simulink model "LQR_sim"  (R2025b)
settings: Solver=VariableStepAuto  StartTime=0.0  StopTime=5  RelTol=1e-3
values from neighbouring files (symbols this model uses):
  A = zeros(4,4)    [get_linearized_matrices.m]
  B = zeros(4,1)    [get_linearized_matrices.m]
  bb = params    [LQR_test.m]
  C = diag([1,0,0,0])    [KalmanFilter.m]    (also in get_linearized_matrices.m = eye(4))
  D = zeros(4,1)    [get_linearized_matrices.m]
  ic = [0; 0.175; 0; 0]    [LQR_test.m]
  K = get_gains_LQR_vertical(0)    [bandwidth_test.m]
  ref = [0;0; 1; 0]    [LQR_test.m]
undefined symbols (not defined in the file or in its folder): Kr
settings Model: Creator=JPham  LastModifiedBy=JPham

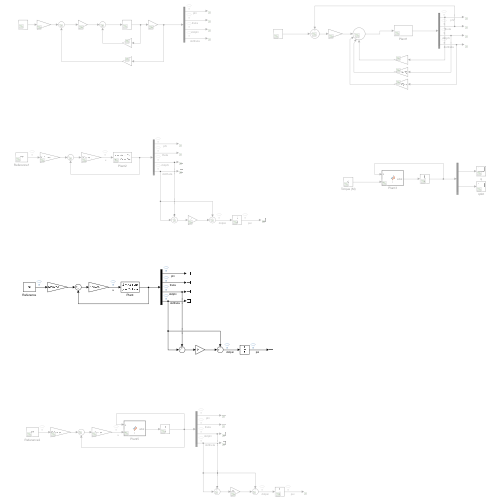
[thumbnail: Simulink's stored preview of the top-level diagram]
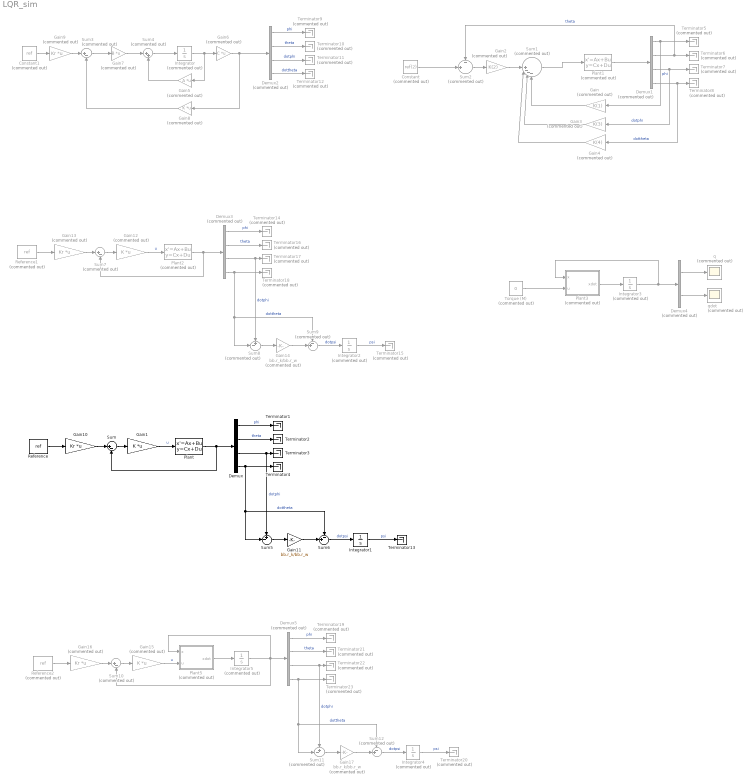
== system LQR_sim ==
  Constant : Constant  Commented=on  Value=ref(2)
  Constant1 : Constant  Commented=on  Value=ref
  Demux : Demux
  Demux{1..3,5} (4 alike) : Demux  Commented=on
  Demux4 : Demux  Commented=on  Outputs=2
  Gain : Gain  Commented=on  Gain=K(1)
  Gain1 : Gain  Gain=K  Multiplication=Matrix(K*u) (u vector)
  Gain10 : Gain  Gain=Kr  Multiplication=Matrix(K*u) (u vector)
  Gain11 : Gain  Gain=bb.r_k/bb.r_w
  Gain12 : Gain  Commented=on  Gain=K  Multiplication=Matrix(K*u) (u vector)
  Gain13 : Gain  Commented=on  Gain=Kr  Multiplication=Matrix(K*u) (u vector)
  Gain14 : Gain  Commented=on  Gain=bb.r_k/bb.r_w
  Gain15 : Gain  Commented=on  Gain=K  Multiplication=Matrix(K*u) (u vector)
  Gain16 : Gain  Commented=on  Gain=Kr  Multiplication=Matrix(K*u) (u vector)
  Gain17 : Gain  Commented=on  Gain=bb.r_k/bb.r_w
  Gain2 : Gain  Commented=on  Gain=K(2)
  Gain3 : Gain  Commented=on  Gain=K(3)
  Gain4 : Gain  Commented=on  Gain=K(4)
  Gain5 : Gain  Commented=on  Gain=A  Multiplication=Matrix(K*u)
  Gain6 : Gain  Commented=on  Gain=C  Multiplication=Matrix(K*u)
  Gain7 : Gain  Commented=on  Gain=B  Multiplication=Matrix(K*u)
  Gain8 : Gain  Commented=on  Gain=K  Multiplication=Matrix(K*u)
  Gain9 : Gain  Commented=on  Gain=Kr  Multiplication=Matrix(K*u)
  Integrator : Integrator  Commented=on  InitialCondition=ic
  Integrator1 : Integrator
  Integrator2 : Integrator  Commented=on
  Integrator3 : Integrator  Commented=on  InitialCondition=[0; 0.3; 0; -1]  ContinuousStateAttributes='angle'
  Integrator4 : Integrator  Commented=on
  Integrator5 : Integrator  Commented=on  InitialCondition=ic  ContinuousStateAttributes='angle'
  Plant : StateSpace  A=A  B=B  C=C  D=D  InitialCondition=ic  ContinuousStateAttributes={'phi', 'theta', 'dot_phi', 'dot_theta'}
  Plant1 : StateSpace  Commented=on  A=A  B=B  C=C  D=D  InitialCondition=ic  ContinuousStateAttributes={'phi', 'theta', 'dot_phi', 'dot_theta'}
  Plant2 : StateSpace  Commented=on  A=A  B=B  C=C  D=D  InitialCondition=ic  ContinuousStateAttributes={'phi', 'theta', 'dot_phi', 'dot_theta'}
  Plant3 : MATLAB Function  Commented=on  TreatAsAtomicUnit=on
  Plant5 : MATLAB Function  Commented=on  TreatAsAtomicUnit=on
  Reference : Constant  Value=ref
  Reference1 : Constant  Commented=on  Value=ref
  Reference2 : Constant  Commented=on  Value=ref
  Sum : Sum  Inputs=|+-
  Sum1 : Sum  Commented=on  Inputs=|||+---
  Sum10 : Sum  Commented=on  Inputs=|+-
  Sum11 : Sum  Commented=on  Inputs=+-|
  Sum12 : Sum  Commented=on  Inputs=-+|
  Sum2 : Sum  Commented=on  Inputs=-|+||
  Sum3 : Sum  Commented=on  Inputs=|+-
  Sum4 : Sum  Commented=on  Inputs=|++
  Sum5 : Sum  Inputs=+-|
  Sum6 : Sum  Inputs=-+|
  Sum7 : Sum  Commented=on  Inputs=|+-
  Sum8 : Sum  Commented=on  Inputs=+-|
  Sum9 : Sum  Commented=on  Inputs=-+|
  Terminator{1..4,13} (5 alike) : Terminator
  Terminator{5..12,14..23} (18 alike) : Terminator  Commented=on
  Torque (M) : Constant  Commented=on  Value=0
  q : Scope  Commented=on
      settings: ActiveDisplayYMinimum=-0.64976  ActiveDisplayYMaximum=0.40553
  qdot : Scope  Commented=on
      settings: ActiveDisplayYMinimum=-1.78097  ActiveDisplayYMaximum=0.83846
  wires:
  Torque (M)/1 -> Plant3/2(u)
  Plant3/1(xdot) -> Integrator3/1
  Integrator3/1 -> Demux4/1, Plant3/1(x)
  Demux4/1 -> q/1
  Gain15/1 -> Plant5/2(u)  "u"
  Demux5/3 -> Terminator22/1, Sum11/1  "dotphi"
  Demux5/2 -> Terminator21/1  "theta"
  Demux5/4 -> Terminator23/1, Sum11/2, Sum12/1  "dottheta"
  Demux5/1 -> Terminator19/1  "phi"
  Sum10/1 -> Gain15/1
  Sum11/1 -> Gain17/1
  Sum12/1 -> Integrator4/1  "dotpsi"
  Reference2/1 -> Gain16/1
  Gain16/1 -> Sum10/1
  Integrator4/1 -> Terminator20/1  "psi"
  Integrator5/1 -> Plant5/1(x), Sum10/2, Demux5/1
  Plant5/1(xdot) -> Integrator5/1
  Sum9/1 -> Integrator2/1  "dotpsi"
  Gain12/1 -> Plant2/1  "u"
  Reference/1 -> Gain10/1
  Gain7/1 -> Sum4/1
  Demux1/2 -> Terminator6/1, Sum2/1  "theta"
  Sum1/1 -> Plant1/1
  Gain1/1 -> Plant/1  "u"
  Sum8/1 -> Gain14/1
  Sum4/1 -> Integrator/1
  Demux1/4 -> Gain4/1, Terminator8/1  "dottheta"
  Demux/1 -> Terminator1/1  "phi"
  Sum5/1 -> Gain11/1
  Gain5/1 -> Sum4/2
  Reference1/1 -> Gain13/1
  Integrator/1 -> Gain5/1, Gain6/1
  Gain14/1 -> Sum9/2
  Demux3/4 -> Terminator18/1, Sum8/2, Sum9/1  "dottheta"
  Demux2/2 -> Terminator10/1  "theta"
  Demux2/4 -> Terminator12/1  "dottheta"
  Sum/1 -> Gain1/1
  Demux4/2 -> qdot/1
  Demux2/3 -> Terminator11/1  "dotphi"
  Gain/1 -> Sum1/4
  Constant/1 -> Sum2/2
  Gain9/1 -> Sum3/1
  Gain4/1 -> Sum1/2
  Plant1/1 -> Demux1/1
  Integrator2/1 -> Terminator15/1  "psi"
  Gain8/1 -> Sum3/2
  Sum3/1 -> Gain7/1
  Sum6/1 -> Integrator1/1  "dotpsi"
  Demux3/3 -> Terminator17/1, Sum8/1  "dotphi"
  Gain3/1 -> Sum1/3
  Demux/3 -> Sum5/1, Terminator3/1  "dotphi"
  Integrator1/1 -> Terminator13/1  "psi"
  Demux/2 -> Terminator2/1  "theta"
  Sum2/1 -> Gain2/1
  Sum7/1 -> Gain12/1
  Demux/4 -> Sum6/1, Sum5/2, Terminator4/1  "dottheta"
  Demux1/1 -> Gain/1, Terminator5/1  "phi"
  Demux1/3 -> Gain3/1, Terminator7/1  "dotphi"
  Gain13/1 -> Sum7/1
  Plant/1 -> Sum/2, Demux/1
  Demux3/2 -> Terminator16/1  "theta"
  Constant1/1 -> Gain9/1
  Demux3/1 -> Terminator14/1  "phi"
  Gain11/1 -> Sum6/2
  Gain6/1 -> Demux2/1, Gain8/1
  Gain17/1 -> Sum12/2
  Plant2/1 -> Demux3/1, Sum7/2
  Demux2/1 -> Terminator9/1  "phi"
  Gain2/1 -> Sum1/1
  Gain10/1 -> Sum/1

== matlab function LQR_sim/Plant3 ==
  data: x input; u input; xdot output; p parameter
function xdot = f(x, u, p)
    % Define dimensions for code generation
    % x is 4x1 state: [phi; theta; phi_dot; theta_dot]
    % u is scalar torque (leave as constant for now)
    % p is the parameter structure, loaded into simulink in Model Explorer
    
    q1  = x(1); % phi
    q2  = x(2); % theta
    q1d = x(3); % phi_dot
    q2d = x(4); % theta_dot
    
    % Aux Parameters
    m_tot = p.m_k + p.m_A + p.m_w;
    r_tot = p.r_k + p.r_w;
    gamma = p.l*p.m_A + (p.r_k + p.r_w)*p.m_w;
    
    % M matrix
    M11 = m_tot*p.r_k^2 + p.Theta_k + (p.r_k/p.r_w)^2 * p.Theta_w;
    M12 = -(p.r_k/p.r_w^2)*r_tot*p.Theta_w + gamma*p.r_k*cos(q2);
    M21 = M12;
    M22 = (r_tot^2/p.r_w^2)*p.Theta_w + p.Theta_A + p.m_A*p.l^2 + p.m_w*r_tot^2;
    
    M = [M11, M12;
         M21, M22];
    
    % C vector
    Cvec = [ -p.r_k*gamma*sin(q2)*q2d^2; 
              0 ];
    % G vector
    Gvec = [ 0; 
            -p.g*sin(q2)*gamma ];
    % S vector (f_NP = S*u(t))
    S = [ p.r_k / p.r_w; -p.r_k / p.r_w ];
    
    % --- Dynamics Calculation ---
    F_np = S * u; 
    
    % Solve for qdd from M * qdd + C + G = F_np
    % qdd = M \ (F_np - C - G) = [theta_doubledot; phi_doubledot]
    qdd = M \ (F_np - Cvec - Gvec);
    
    % Assemble xdot
    xdot = [q1d;
            q2d;
            qdd(1);
            qdd(2)];
end

== matlab function LQR_sim/Plant5 ==
  data: x input; u input; xdot output
function xdot = f(x, u)
    % Define dimensions for code generation
    % x is 4x1 state: [phi; theta; phi_dot; theta_dot]
    % u is scalar torque (leave as constant for now)
    % p is the parameter structure, loaded into simulink in Model Explorer
    
    q1  = x(1); % phi
    q2  = x(2); % theta
    q1d = x(3); % phi_dot
    q2d = x(4); % theta_dot
    
    p = params;
    % Aux Parameters
    m_tot = p.m_k + p.m_A + p.m_w;
    r_tot = p.r_k + p.r_w;
    gamma = p.l*p.m_A + (p.r_k + p.r_w)*p.m_w;
    
    % M matrix
    M11 = m_tot*p.r_k^2 + p.Theta_k + (p.r_k/p.r_w)^2 * p.Theta_w;
    M12 = -(p.r_k/p.r_w^2)*r_tot*p.Theta_w + gamma*p.r_k*cos(q2);
    M21 = M12;
    M22 = (r_tot^2/p.r_w^2)*p.Theta_w + p.Theta_A + p.m_A*p.l^2 + p.m_w*r_tot^2;
    
    M = [M11, M12;
         M21, M22];
    
    % C vector
    Cvec = [ -p.r_k*gamma*sin(q2)*q2d^2; 
              0 ];
    % G vector
    Gvec = [ 0; 
            -p.g*sin(q2)*gamma ];
    % S vector (f_NP = S*u(t))
    S = [ p.r_k / p.r_w; -p.r_k / p.r_w ];
    
    % --- Dynamics Calculation ---
    F_np = S * u; 
    
    % Solve for qdd from M * qdd + C + G = F_np
    % qdd = M \ (F_np - C - G) = [theta_doubledot; phi_doubledot]
    qdd = M \ (F_np - Cvec - Gvec);
    
    % Assemble xdot
    xdot = [q1d;
            q2d;
            qdd(1);
            qdd(2)];
end
